simulink model "sensor_fault_profiles"  (Simulink 7.9)
settings: Solver=ode45  StartTime=0.0  StopTime=10.0  RelTol=1e-3
values from neighbouring files (symbols this model uses):
  a_slope = -0.6    [check_time_with_lqg_and_nn.m]    (also in current_inc_abr.m; fault_tests_abrupt_add_igva_iFD.m = 20; fault_tests_abrupt_add_igva_lqgFD.m = 20; fault_tests_abrupt_bias_igva_iFD.m)
  acceleration_fault_time = 7    [check_time_with_lqg_and_nn.m]    (also in current_inc_abr.m; fault_tests_abrupt_add_igva_iFD.m = 0.5; fault_tests_abrupt_add_igva_lqgFD.m = 0.5; fault_tests_abrupt_bias_igva_iFD.m = 0.5)
  current_fault_time = 7    [check_time_with_lqg_and_nn.m]    (also in current_inc_abr.m = 1; fault_tests_abrupt_add_igva_iFD.m = 2; fault_tests_abrupt_add_igva_lqgFD.m = 2; fault_tests_abrupt_bias_igva_iFD.m = 2)
  fault_type_a = 1    [check_time_with_lqg_and_nn.m]    (also in current_inc_abr.m; fault_tests_abrupt_add_igva_iFD.m = 2; fault_tests_abrupt_add_igva_lqgFD.m = 2; fault_tests_abrupt_bias_igva_iFD.m = 5)
  fault_type_i = 1    [check_time_with_lqg_and_nn.m]    (also in current_inc_abr.m = 2; fault_tests_abrupt_add_igva_iFD.m = 2; fault_tests_abrupt_add_igva_lqgFD.m = 2; fault_tests_abrupt_bias_igva_iFD.m = 5)
  fault_type_v = 1    [check_time_with_lqg_and_nn.m]    (also in current_inc_abr.m; fault_tests_abrupt_add_igva_iFD.m = 2; fault_tests_abrupt_add_igva_lqgFD.m = 2; fault_tests_abrupt_bias_igva_iFD.m = 5)
  Tsamp = 0.001    [LSDP_controllers_nntraining_data_igva.m]    (also in initialize_LSDP_controllers_igva.m)
  v_slope = -0.6    [check_time_with_lqg_and_nn.m]    (also in current_inc_abr.m; fault_tests_abrupt_add_igva_iFD.m = 0.5; fault_tests_abrupt_add_igva_lqgFD.m = 0.5; fault_tests_abrupt_bias_igva_iFD.m)
  velocity_fault_time = 7    [check_time_with_lqg_and_nn.m]    (also in current_inc_abr.m; fault_tests_abrupt_add_igva_iFD.m = 1.5; fault_tests_abrupt_add_igva_lqgFD.m = 1.5; fault_tests_abrupt_bias_igva_iFD.m = 1.5)
libraries: simulink x9
settings Model: Creator=kostas  LastModifiedBy=kostas

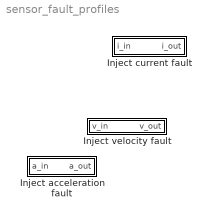
== system sensor_fault_profiles ==
  Inject acceleration fault : Subsystem
  Inject current fault : Subsystem
  Inject velocity fault : Subsystem

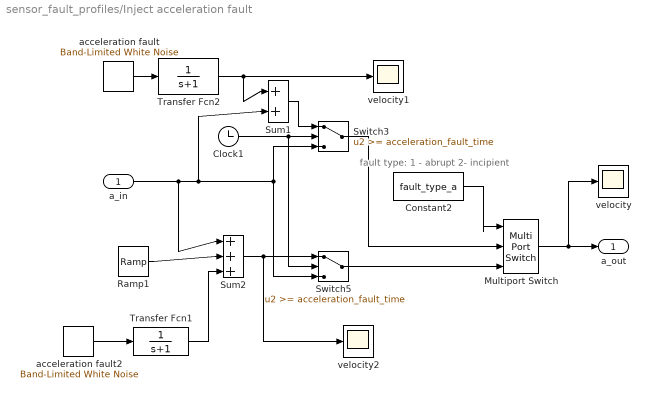
== system sensor_fault_profiles/Inject acceleration fault ==
  note: fault type:
      | 1 - abrupt
      | 2- incipient
  a_in : Inport
  Clock1 : Clock
  Constant2 : Constant  Value=fault_type_a
  Multiport Switch : MultiPortSwitch  Inputs=2  zeroidx=off
  Ramp1 : simulink/Sources/Ramp  slope=a_slope  start=acceleration_fault_time  X0=0
  Sum1 : Sum  Inputs=|++
  Sum2 : Sum  Inputs=|+++
  Switch3 : Switch  Threshold=acceleration_fault_time
  Switch5 : Switch  Threshold=acceleration_fault_time
  Transfer Fcn1 : TransferFcn  Denominator=[1 1]
  Transfer Fcn2 : TransferFcn  Denominator=[1 1]
  acceleration fault : simulink/Sources/Band-Limited White Noise  Cov=0.2  Ts=Tsamp  seed=[23341]
  acceleration fault2 : simulink/Sources/Band-Limited White Noise  Cov=0.01  Ts=Tsamp  seed=[23341]
  velocity : Scope
      settings: TimeRange=6  YMin=0.25  YMax=3.25  SaveName=ScopeData16
  velocity1 : Scope
      settings: TimeRange=6  YMin=0.25  YMax=3.25  SaveName=ScopeData17
  velocity2 : Scope
      settings: TimeRange=5  YMin=-0.05  YMax=0.9  SaveName=ScopeData26
  a_out : Outport
  wires:
  a_in/1 -> Sum2/1, Switch3/3, Switch5/3, Sum1/2
  Clock1/1 -> Switch3/2, Switch5/2
  Transfer Fcn2/1 -> velocity1/1, Sum1/1
  acceleration fault/1 -> Transfer Fcn2/1
  Ramp1/1 -> Sum2/2
  Multiport Switch/1 -> a_out/1, velocity/1
  Switch3/1 -> Multiport Switch/2
  Switch5/1 -> Multiport Switch/3
  Constant2/1 -> Multiport Switch/1
  Sum2/1 -> Switch5/1, velocity2/1
  Sum1/1 -> Switch3/1
  acceleration fault2/1 -> Transfer Fcn1/1
  Transfer Fcn1/1 -> Sum2/3

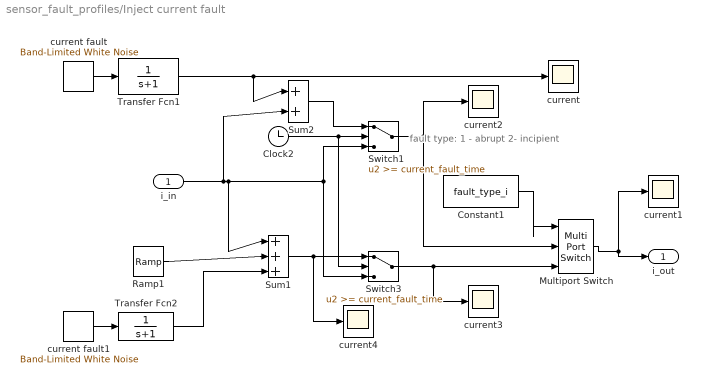
== system sensor_fault_profiles/Inject current fault ==
  note: fault type:
      | 1 - abrupt
      | 2- incipient
  i_in : Inport
  Clock2 : Clock
  Constant1 : Constant  Value=fault_type_i
  Multiport Switch : MultiPortSwitch  Inputs=2  zeroidx=off
  Ramp1 : simulink/Sources/Ramp  slope=4  start=current_fault_time  X0=0
  Sum1 : Sum  Inputs=|+++
  Sum2 : Sum  Inputs=|++
  Switch1 : Switch  Threshold=current_fault_time
  Switch3 : Switch  Threshold=current_fault_time
  Transfer Fcn1 : TransferFcn  Denominator=[1 1]
  Transfer Fcn2 : TransferFcn  Denominator=[1 1]
  current{,1..4} (5 alike) : Scope
      current settings: TimeRange=6  YMin=0.25  YMax=3.25  SaveName=ScopeData15
      current1 settings: TimeRange=7  YMin=-15  YMax=10  SaveName=ScopeData14
      current2 settings: TimeRange=6  YMin=0.25  YMax=3.25  SaveName=ScopeData9
      current3 settings: TimeRange=6  YMin=0.25  YMax=3.25  SaveName=ScopeData23
      current4 settings: TimeRange=2  YMin=2.051319648093839  YMax=8.051319648093839  SaveName=ScopeData24
  current fault : simulink/Sources/Band-Limited White Noise  Cov=1  Ts=Tsamp  seed=[23341]
  current fault1 : simulink/Sources/Band-Limited White Noise  Cov=1  Ts=Tsamp  seed=[23341]
  i_out : Outport
  wires:
  i_in/1 -> Switch1/3, Switch3/3, Sum1/1, Sum2/2
  Clock2/1 -> Switch1/2, Switch3/2
  Transfer Fcn1/1 -> current/1, Sum2/1
  current fault/1 -> Transfer Fcn1/1
  Multiport Switch/1 -> i_out/1, current1/1
  Switch1/1 -> Multiport Switch/2, current2/1
  Constant1/1 -> Multiport Switch/1
  Sum1/1 -> Switch3/1, current4/1
  Switch3/1 -> Multiport Switch/3, current3/1
  Ramp1/1 -> Sum1/2
  Sum2/1 -> Switch1/1
  current fault1/1 -> Transfer Fcn2/1
  Transfer Fcn2/1 -> Sum1/3

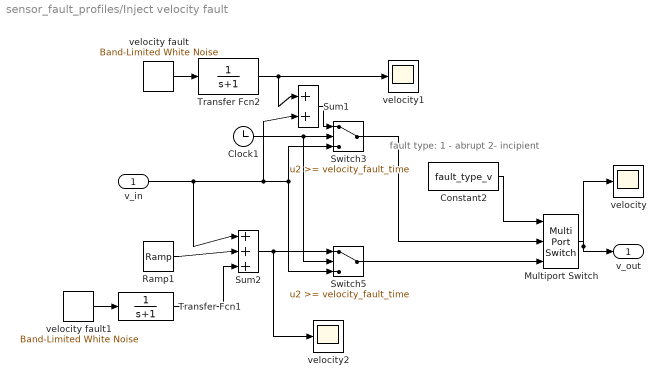
== system sensor_fault_profiles/Inject velocity fault ==
  note: fault type:
      | 1 - abrupt
      | 2- incipient
  v_in : Inport
  Clock1 : Clock
  Constant2 : Constant  Value=fault_type_v
  Multiport Switch : MultiPortSwitch  Inputs=2  zeroidx=off
  Ramp1 : simulink/Sources/Ramp  slope=v_slope  start=velocity_fault_time  X0=0
  Sum1 : Sum  Inputs=|++
  Sum2 : Sum  Inputs=|+++
  Switch3 : Switch  Threshold=velocity_fault_time
  Switch5 : Switch  Threshold=velocity_fault_time
  Transfer Fcn1 : TransferFcn  Denominator=[1 1]
  Transfer Fcn2 : TransferFcn  Denominator=[1 1]
  velocity : Scope
      settings: TimeRange=6  YMin=0.25  YMax=3.25  SaveName=ScopeData19
  velocity fault : simulink/Sources/Band-Limited White Noise  Cov=0.05  Ts=Tsamp  seed=[21342]
  velocity fault1 : simulink/Sources/Band-Limited White Noise  Cov=0.02  Ts=Tsamp  seed=[23341]
  velocity1 : Scope
      settings: TimeRange=6  YMin=0.25  YMax=3.25  SaveName=ScopeData18
  velocity2 : Scope
      settings: TimeRange=6  YMin=0.25  YMax=3.25  SaveName=ScopeData25
  v_out : Outport
  wires:
  v_in/1 -> Sum2/1, Switch3/3, Switch5/3, Sum1/2
  Clock1/1 -> Switch3/2, Switch5/2
  Transfer Fcn2/1 -> velocity1/1, Sum1/1
  velocity fault/1 -> Transfer Fcn2/1
  Ramp1/1 -> Sum2/2
  Multiport Switch/1 -> v_out/1, velocity/1
  Switch3/1 -> Multiport Switch/2
  Switch5/1 -> Multiport Switch/3
  Constant2/1 -> Multiport Switch/1
  Sum2/1 -> Switch5/1, velocity2/1
  Sum1/1 -> Switch3/1
  velocity fault1/1 -> Transfer Fcn1/1
  Transfer Fcn1/1 -> Sum2/3
